simulink model "HevP4OptimalController"  (R2023b)
settings: Solver=FixedStepDiscrete  StartTime=0  StopTime=inf  FixedStep=0.01  RelTol=1e-3  EnableMultiTasking=on
model workspace (MAT data in the model file):
  AccPwrbp = Simulink.Parameter
  AccPwrbp.Value = [0 0]
  AccPwrbp.DataType = 'double'
  AccPwrbp.Complexity = 'real'
  AccPwrbp.Dimensions = [1 2]
  AccSpdbp = Simulink.Parameter
  AccSpdbp.Value = [300 750]
  AccSpdbp.DataType = 'double'
  AccSpdbp.Complexity = 'real'
  AccSpdbp.Dimensions = [1 2]
  BattChrgPwrMax = Simulink.Parameter
  BattChrgPwrMax.Value = -30000
  BattChrgPwrMax.DataType = 'double'
  BattChrgPwrMax.Complexity = 'real'
  BattChrgPwrMax.Dimensions = [1 1]
  BattCurrMax = Simulink.Parameter
  BattCurrMax.Value = 150
  BattCurrMax.DataType = 'double'
  BattCurrMax.Complexity = 'real'
  BattCurrMax.Dimensions = [1 1]
  BattDischrgPwrMax = Simulink.Parameter
  BattDischrgPwrMax.Value = 46000
  BattDischrgPwrMax.DataType = 'double'
  BattDischrgPwrMax.Complexity = 'real'
  BattDischrgPwrMax.Dimensions = [1 1]
  BattTempBp = Simulink.Parameter
  BattTempBp.Value = [243.1 253.1 263.1 273.1 283.1 298.1 313.1]
  BattTempBp.DataType = 'double'
  BattTempBp.Complexity = 'real'
  BattTempBp.Dimensions = [1 7]
  BrkPrsMax = Simulink.Parameter
  BrkPrsMax.Value = 8273709
  BrkPrsMax.DataType = 'double'
  BrkPrsMax.Complexity = 'real'
  BrkPrsMax.Dimensions = [1 1]
  CapLUTBp = Simulink.Parameter
  CapLUTBp.Value = [0 0.01 0.02 0.03 0.04 0.05 0.06 0.07 0.08 0.09 0.1 0.11 0.12 0.13 0.14 0.15 0.16 0.17 0.18 0.19 0.2 0.21 0.22 0.23 0.24 0.25 0.26 0.27 0.28 0.29 0.3 0.31 0.32 0.33 0.34 0.35 0.36 0.37 0.38 0.39 0.4 0.41 0.42 0.43 0.44 0.45 0.46 0.47 0.48 0.49 0.5 0.51 0.52 0.53 0.54 0.55 0.56 0.57 0.58 0.59 0.6 0.61 0.62 0.63 0.64 0.65 0.66 0.67 0.68 0.69 0.7 0.71 0.72 0.73 0.74 0.75 0.76 0.77 0.78 0.79 0.8 0.81 0.82 0.83 0.84 0.85 0.86 0.87 0.88 0.89 0.9 0.91 0.92 0.93 0.94 0.95 0.96 0.97 0.98 0.99 1]
  CapLUTBp.DataType = 'double'
  CapLUTBp.Complexity = 'real'
  CapLUTBp.Dimensions = [1 101]
  CapSOCBp = Simulink.Parameter
  CapSOCBp.Value = [0 0.2 0.4 0.6 0.8 1]
  CapSOCBp.DataType = 'double'
  CapSOCBp.Complexity = 'real'
  CapSOCBp.Dimensions = [1 6]
  ChrgLmt_bpt = Simulink.Parameter
  ChrgLmt_bpt.Value = [1 1 1 1 1 1 1 0.9 0.7 0.5 0]
  ChrgLmt_bpt.DataType = 'double'
  ChrgLmt_bpt.Complexity = 'real'
  ChrgLmt_bpt.Dimensions = [1 11]
  DischrgLmt_bpt = Simulink.Parameter
  DischrgLmt_bpt.Value = [0 0.5 0.7 0.9 1 1 1 1 1 1 1]
  DischrgLmt_bpt.DataType = 'double'
  DischrgLmt_bpt.Complexity = 'real'
  DischrgLmt_bpt.Dimensions = [1 11]
  ECMS_Ki = Simulink.Parameter
  ECMS_Ki.Value = 0.1
  ECMS_Ki.DataType = 'double'
  ECMS_Ki.Complexity = 'real'
  ECMS_Ki.Dimensions = [1 1]
  ECMS_Kp = Simulink.Parameter
  ECMS_Kp.Value = 3
  ECMS_Kp.DataType = 'double'
  ECMS_Kp.Complexity = 'real'
  ECMS_Kp.Dimensions = [1 1]
  ECMS_method = Simulink.Parameter
  ECMS_method.Value = 1
  ECMS_method.DataType = 'double'
  ECMS_method.Complexity = 'real'
  ECMS_method.Dimensions = [1 1]
  ECMS_s = Simulink.Parameter
  ECMS_s.Value = 3.65
  ECMS_s.DataType = 'double'
  ECMS_s.Complexity = 'real'
  ECMS_s.Dimensions = [1 1]
  Em = Simulink.Parameter
  Em.Value = [2.8 3.228 3.284 3.361 3.408 3.427 3.472 3.477 3.493 3.504 3.516 3.528 3.537 3.545 3.555 3.561 3.566 3.576 3.587 3.589 3.594 3.6 3.608 3.61 3.616 3.619 3.626 3.632 3.637 3.64 3.645 3.646 3.652 3.655 3.658 3.661 3.664 3.668 3.673 3.678 3.68 3.681 3.686 3.692 3.699 3.702 3.705 3.71 3.717 3.723 3.728 3.733 3.735 3.742 3.749 3.755 3.761 3.768 3.773 3.78 3.791 3.798 3.798 3.814 3.818 3.825 3.841 3.846 3.855 3.863 3.877 3.885 3.894 3.907 3.919 3.926 3.935 3.944 3.954 3.964 3.974 3.988 3.998 4.014 4.029 4.034 4.047 4.065 4.074 4.086 4.097 4.131 4.126 4.138 4.15 4.18 4.174 4.187 4.207 4.231 4.221]
  Em.DataType = 'double'
  Em.Complexity = 'real'
  Em.Dimensions = [1 101]
  G = Simulink.Parameter
  G.Value = [0 1 2 3 4 5 6]
  G.DataType = 'double'
  G.Complexity = 'real'
  G.Dimensions = [1 7]
  HEVEngTrq_min = Simulink.Parameter
  HEVEngTrq_min.Value = 16.186104388
  HEVEngTrq_min.DataType = 'double'
  HEVEngTrq_min.Complexity = 'real'
  HEVEngTrq_min.Dimensions = [1 1]
  Lhv = Simulink.Parameter
  Lhv.Value = 46000000
  Lhv.DataType = 'double'
  Lhv.Complexity = 'real'
  Lhv.Dimensions = [1 1]
  N = Simulink.Parameter
  N.Value = [1 4.212 2.637 1.8 1.386 1 0.772]
  N.DataType = 'double'
  N.Complexity = 'real'
  N.Dimensions = [1 7]
  N_P0 = 0.001
  N_idle = Simulink.Parameter
  N_idle.Value = 750
  N_idle.DataType = 'double'
  N_idle.Complexity = 'real'
  N_idle.Dimensions = [1 1]
  Ndiff = Simulink.Parameter
  Ndiff.Value = 3.32
  Ndiff.DataType = 'double'
  Ndiff.Complexity = 'real'
  Ndiff.Dimensions = [1 1]
  Ndiff_P4 = Simulink.Parameter
  Ndiff_P4.Value = 4.1
  Ndiff_P4.DataType = 'double'
  Ndiff_P4.Complexity = 'real'
  Ndiff_P4.Dimensions = [1 1]
  Ngrid = Simulink.Parameter
  Ngrid.Value = 200
  Ngrid.DataType = 'double'
  Ngrid.Complexity = 'real'
  Ngrid.Dimensions = [1 1]
  Np = Simulink.Parameter
  Np.Value = 1
  Np.DataType = 'double'
  Np.Complexity = 'real'
  Np.Dimensions = [1 1]
  Ns = Simulink.Parameter
  Ns.Value = 72
  Ns.DataType = 'double'
  Ns.Complexity = 'real'
  Ns.Dimensions = [1 1]
  PenaltyFctr = Simulink.Parameter
  PenaltyFctr.Value = 10000000
  PenaltyFctr.DataType = 'double'
  PenaltyFctr.Complexity = 'real'
  PenaltyFctr.Dimensions = [1 1]
  RInt = Simulink.Parameter
  RInt.Value = [0.008846  0.009319  0.009027  0.00847  0.01032  0.01314; 0.006389  0.006554  0.005553  0.005525  0.006043  0.007805; 0.004364  0.004101  0.00406  0.003452  0.003846  0.004517; 0.002031  0.002563  0.002532  0.00246  0.002716  0.003047; 0.001443  0.001825  0.001795  0.001778  0.001924  0.002234; 0.0005603  0.0007192  0.0006887  0.0007557  0.0007355  0.001014; 0.001028  0.001338  0.001  0.001536  0.001546  0.002789]
  RInt.DataType = 'double'
  RInt.Complexity = 'real'
  RInt.Dimensions = [7 6]
  Re = Simulink.Parameter
  Re.Value = 0.327
  Re.DataType = 'double'
  Re.Complexity = 'real'
  Re.Dimensions = [1 1]
  RegenBrkCutOff = Simulink.Parameter
  RegenBrkCutOff.Value = [0 1]
  RegenBrkCutOff.DataType = 'double'
  RegenBrkCutOff.Complexity = 'real'
  RegenBrkCutOff.Dimensions = [1 2]
  RegenBrkSpd_bpt = Simulink.Parameter
  RegenBrkSpd_bpt.Value = [2.2352 4.4704]
  RegenBrkSpd_bpt.DataType = 'double'
  RegenBrkSpd_bpt.Complexity = 'real'
  RegenBrkSpd_bpt.Dimensions = [1 2]
  Rm = Simulink.Parameter
  Rm.Value = 0.15
  Rm.DataType = 'double'
  Rm.Complexity = 'real'
  Rm.Dimensions = [1 1]
  SOCTrgt = Simulink.Parameter
  SOCTrgt.Value = 60
  SOCTrgt.DataType = 'double'
  SOCTrgt.Complexity = 'real'
  SOCTrgt.Dimensions = [1 1]
  SOC_bpt = Simulink.Parameter
  SOC_bpt.Value = [0 0.1 0.2 0.3 0.4 0.5 0.6 0.7 0.8 0.9 1]
  SOC_bpt.DataType = 'double'
  SOC_bpt.Complexity = 'real'
  SOC_bpt.Dimensions = [1 11]
  SOCmax = Simulink.Parameter
  SOCmax.Value = 80
  SOCmax.DataType = 'double'
  SOCmax.Complexity = 'real'
  SOCmax.Dimensions = [1 1]
  SOCmin = Simulink.Parameter
  SOCmin.Value = 40
  SOCmin.DataType = 'double'
  SOCmin.Complexity = 'real'
  SOCmin.Dimensions = [1 1]
  T = Simulink.Parameter
  T.Value = 300
  T.DataType = 'double'
  T.Complexity = 'real'
  T.Dimensions = [1 1]
  T_eff_bp = Simulink.Parameter
  T_eff_bp.Value = [0 20 40 60 80 100 120 140 160 180 200]
  T_eff_bp.DataType = 'double'
  T_eff_bp.Complexity = 'real'
  T_eff_bp.Dimensions = [1 11]
  T_eff_bp_P0 = Simulink.Parameter
  T_eff_bp_P0.Value = [5.30516476973 5.78745247607 6.36619772368 7.07355302631 7.95774715459 9.09456817668 10.6103295395 12.7323954474 15.9154943092 21.2206590789 66.6666666667]
  T_eff_bp_P0.DataType = 'double'
  T_eff_bp_P0.Complexity = 'real'
  T_eff_bp_P0.Dimensions = [1 11]
  T_t = Simulink.Parameter
  T_t.Value = [200 200 200 200 190.9859317 143.2394488 114.591559 95.49296586 81.85111359 71.61972439 63.66197724 57.29577951 52.08707228 47.74648293]
  T_t.DataType = 'double'
  T_t.Complexity = 'real'
  T_t.Dimensions = [1 14]
  T_t_P0 = Simulink.Parameter
  T_t_P0.Value = [66.6666666667 66.6666666667 66.6666666667 66.6666666667 21.2206590789 15.9154943092 12.7323954474 10.6103295395 9.09456817668 7.95774715459 7.07355302631 6.36619772368 5.78745247607 5.30516476973]
  T_t_P0.DataType = 'double'
  T_t_P0.Complexity = 'real'
  T_t_P0.Dimensions = [1 14]
  Temp_bpts = Simulink.Parameter
  Temp_bpts.Value = [313 358]
  Temp_bpts.DataType = 'double'
  Temp_bpts.Complexity = 'real'
  Temp_bpts.Dimensions = [1 2]
  TracPenaltyFctr = Simulink.Parameter
  TracPenaltyFctr.Value = 50
  TracPenaltyFctr.DataType = 'double'
  TracPenaltyFctr.Complexity = 'real'
  TracPenaltyFctr.Dimensions = [1 1]
  Trq_bpts = Simulink.Parameter
  Trq_bpts.Value = [25 50 75 100 150 200 250]
  Trq_bpts.DataType = 'double'
  Trq_bpts.Complexity = 'real'
  Trq_bpts.Dimensions = [1 7]
  a = Simulink.Parameter
  a.Value = 3
  a.DataType = 'double'
  a.Complexity = 'real'
  a.Dimensions = [1 1]
  disk_abore = Simulink.Parameter
  disk_abore.Value = 0.05
  disk_abore.DataType = 'double'
  disk_abore.Complexity = 'real'
  disk_abore.Dimensions = [1 1]
  eff = Simulink.Parameter
  eff.Value = 98
  eff.DataType = 'double'
  eff.Complexity = 'real'
  eff.Dimensions = [1 1]
  efficiency_table = Simulink.Parameter
  efficiency_table.Value = [0.52  0.78  0.8  0.82  0.82  0.8  0.78  0.78  0.76  0.74  0.7; 0.52  0.78  0.8  0.82  0.82  0.8  0.78  0.78  0.76  0.74  0.7; 0.52  0.78  0.84  0.86  0.86  0.86  0.86  0.84  0.84  0.82  0.82; 0.52  0.8  0.86  0.86  0.88  0.88  0.88  0.86  0.86  0.84  0.84; 0.52  0.8  0.86  0.88  0.88  0.88  0.88  0.88  0.86  0.86  0.86; 0.52  0.8  0.86  0.88  0.9  0.9  0.9  0.9  0.88  0.88  0.88; 0.52  0.82  0.88  0.9  0.91  0.91  0.92  0.92  0.92  0.91  0.91; 0.52  0.82  0.88  0.91  0.91  0.92  0.93  0.93  0.93  0.93  0.93; 0.52  0.84  0.9  0.92  0.92  0.93  0.93  0.93  0.93  0.93  0.93; 0.62  0.86  0.91  0.93  0.93  0.93  0.93  0.93  0.93  0.93  0.93; 0.66  0.86  0.91  0.93  0.93  0.93  0.93  0.93  0.93  0.93  0.93; 0.7  0.86  0.92  0.93  0.93  0.93  0.93  0.93  0.93  0.93  0.93; 0.7  0.86  0.92  0.93  0.93  0.93  0.93  0.93  0.93  0.93  0.93; 0.72  0.86  0.91  0.93  0.93  0.93  0.93  0.93  0.93  0.93  0.93]
  efficiency_table.DataType = 'double'
  efficiency_table.Complexity = 'real'
  efficiency_table.Dimensions = [14 11]
  eta = Simulink.Parameter
  eta.Value = 1
  eta.DataType = 'double'
  eta.Complexity = 'real'
  eta.Dimensions = [1 1]
  eta_dcdc = Simulink.Parameter
  eta_dcdc.Value = 0.98
  eta_dcdc.DataType = 'double'
  eta_dcdc.Complexity = 'real'
  eta_dcdc.Dimensions = [1 1]
  eta_diff = Simulink.Parameter
  eta_diff.Value = 0.98
  eta_diff.DataType = 'double'
  eta_diff.Complexity = 'real'
  eta_diff.Dimensions = [1 1]
  eta_tbl = Simulink.Parameter
  eta_tbl.Value = [1 1 1 1 1 1 1 1 1 1 1 1 ... (1078 elements, 7x11x7x2)]
  eta_tbl.DataType = 'double'
  eta_tbl.Complexity = 'real'
  eta_tbl.Dimensions = [7 11 7 2]
  f_fuel = Simulink.Parameter
  f_fuel.Value = [0 0 0 0 0 0 0 0 0 0 0 0 ... (256 elements, 16x16)]
  f_fuel.DataType = 'double'
  f_fuel.Complexity = 'real'
  f_fuel.Dimensions = [16 16]
  f_tbrake = Simulink.Parameter
  f_tbrake.Value = [0 15 15 15 15 15 15 15 15 15 15 15 ... (256 elements, 16x16)]
  f_tbrake.DataType = 'double'
  f_tbrake.Complexity = 'real'
  f_tbrake.Dimensions = [16 16]
  f_tbrake_min = Simulink.Parameter
  f_tbrake_min.Value = [0 6.47839451267 6.81037951773 6.98724865221 7.21080756514 7.41442983108 7.6087152853 7.78836492927 7.96107212367 8.10510304828 8.24671964745 8.36469696542 8.49674350738 8.62005140167 8.74715716666 8.88039047922]
  f_tbrake_min.DataType = 'double'
  f_tbrake_min.Complexity = 'real'
  f_tbrake_min.Dimensions = [1 16]
  f_tbrake_n_bpt = Simulink.Parameter
  f_tbrake_n_bpt.Value = [0 750 1053.57142857 1357.14285714 1660.71428571 1964.28571429 2267.85714286 2571.42857143 2875 3178.57142857 3482.14285714 3785.71428571 4089.28571429 4392.85714286 4696.42857143 5000]
  f_tbrake_n_bpt.DataType = 'double'
  f_tbrake_n_bpt.Complexity = 'real'
  f_tbrake_n_bpt.Dimensions = [1 16]
  f_tbrake_t_bpt = Simulink.Parameter
  f_tbrake_t_bpt.Value = [0 15 26.4285714286 37.8571428571 49.2857142857 60.7142857143 72.1428571429 83.5714285714 95 106.428571429 117.857142857 129.285714286 140.714285714 152.142857143 163.571428571 175]
  f_tbrake_t_bpt.DataType = 'double'
  f_tbrake_t_bpt.Complexity = 'real'
  f_tbrake_t_bpt.Dimensions = [1 16]
  mu_kinetic = Simulink.Parameter
  mu_kinetic.Value = 0.35
  mu_kinetic.DataType = 'double'
  mu_kinetic.Complexity = 'real'
  mu_kinetic.Dimensions = [1 1]
  num_pads = Simulink.Parameter
  num_pads.Value = 2
  num_pads.DataType = 'double'
  num_pads.Complexity = 'real'
  num_pads.Dimensions = [1 1]
  omega_bpts = Simulink.Parameter
  omega_bpts.Value = [500.383141081 749.619781963 1002.67614148 1250.9578527 1499.23956393 1747.52127515 1995.80298637 2501.9157054 2998.47912785 4001.15526933 5003.83141081]
  omega_bpts.DataType = 'double'
  omega_bpts.Complexity = 'real'
  omega_bpts.Dimensions = [1 11]
  w_eff_bp = Simulink.Parameter
  w_eff_bp.Value = [0 500 1000 1432.391138 1500 2000 2500 3000 3500 4000 4500 5000 5500 6000]
  w_eff_bp.DataType = 'double'
  w_eff_bp.Complexity = 'real'
  w_eff_bp.Dimensions = [1 14]
  w_eff_bp_P0 = Simulink.Parameter
  w_eff_bp_P0.Value = [0 500 1000 1432.39448783 4500 6000 7500 9000 10500 12000 13500 15000 16500 18000]
  w_eff_bp_P0.DataType = 'double'
  w_eff_bp_P0.Complexity = 'real'
  w_eff_bp_P0.Dimensions = [1 14]
libraries: simulink x3, autolibhevctrlrcommon x2, autolibhevctrlr x1
settings Model: DataDictionary=HevP4OptimalController.sldd  ModifiedByFormat=The MathWorks, Inc.  Creator=The MathWorks, Inc.  LastModifiedBy=The MathWorks, Inc.
settings SolverCC: AlgebraicLoopSolver=TrustRegion  MaxZcPerStep=1
settings DataIOCC: SaveOutput=off  SignalLogging=off  DSMLogging=off  SaveTime=off  ReturnWorkspaceOutputs=off
settings OptimizationCC: DefaultParameterBehavior=Inlined  EnhancedBackFolding=on  PassReuseOutputArgsAs=Individual arguments  ZeroExternalMemoryAtStartup=off  ZeroInternalMemoryAtStartup=off  EfficientMapNaN2IntZero=off  OptimizeBlockOrder=speed  DifferentSizesBufferReuse=on  OptimizationCustomize=off  EfficientTunableParamExpr=on
settings DebuggingCC: UnderspecifiedInitializationDetection=Classic  MergeDetectMultiDrivingBlocksExec=none  ParameterTunabilityLossMsg=error  UnconnectedInputMsg=warning  UnconnectedOutputMsg=warning  UnconnectedLineMsg=warning  SubsystemReferenceDiagnosticForUnitTest=warning  SFUnusedDataAndEventsDiag=none  ArithmeticOperatorsInVariantConditions=warning
settings HardwareCC: TargetBitPerPointer=64  TargetBitPerSizeT=64  TargetBitPerPtrDiffT=64  TargetLongLongMode=on  TargetIntDivRoundTo=Zero  TargetEndianess=LittleEndian  TargetWordSize=64  TargetHWDeviceType=MATLAB Host  ProdEqTarget=off
settings ModelReferenceCC: EnableRefExpFcnMdlSchedulingChecks=on
settings SFSimCC: SimUseLocalCustomCode=off  SimGenImportedTypeDefs=on  MATLABDynamicMemAlloc=off
settings RTWCC: Description=AUTOSAR  SystemTargetFile=autosar.tlc  GenCodeOnly=on  TemplateMakefile=ert_default_tmf  RTWUseLocalCustomCode=off  DLArmComputeVersion=19.05
settings CodeAppCC: ForceParamTrailComments=on  IgnoreCustomStorageClasses=off  MaxIdLength=128  OperatorAnnotations=on  SimulinkDataObjDesc=on  SFDataObjDesc=on  InsertBlockDesc=on
settings STFCustomTargetCC: TargetLangStandard=C89/C90 (ANSI)  MultiwordLength=256  ParMdlRefBuildCompliant=on  CompOptLevelCompliant=on  IncludeMdlTerminateFcn=off  CombineOutputUpdateFcns=on  SuppressErrorStatus=on  ERTCustomFileBanners=on  SupportNonFinite=off  SupportComplex=off  SupportContinuousTime=off  SupportNonInlinedSFcns=off  RemoveResetFunc=on  MATLABClassNameForMDSCustomization=Simulink.SoftwareTarget.ERTCustomization  AutosarCompliant=on  UseToolchainInfoCompliant=on  LookupTableObjectStructAxisOrder=2,1,3,4,...  LUTObjectStructOrderEvenSpacing=Size,Table,Breakpoints  SystemTargetFile=autosar.tlc
settings ERTTargetCC: ConcurrentExecutionCompliant=off  IncludeMdlTerminateFcn=off  SuppressErrorStatus=on  SupportNonFinite=off  SupportComplex=off  ModelStepFunctionPrototypeControlCompliant=off  CPPClassGenCompliant=off  AutosarCompliant=on  LookupTableObjectStructAxisOrder=2,1,3,4,...  LUTObjectStructOrderEvenSpacing=Size,Table,Breakpoints  InlinedParameterPlacement=NonHierarchical  ERTCustomFileTemplate=example_file_process.tlc
settings ConfigComp: CovMetricSettings=dsw  CovSaveCumulativeToWorkspaceVar=on  CovSaveSingleToWorkspaceVar=on  CovExternalEMLEnable=off

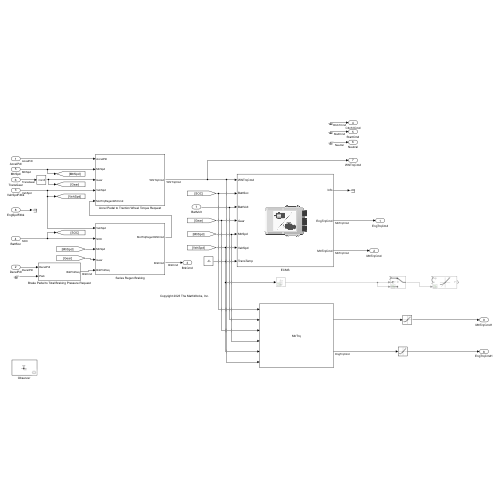
[thumbnail: Simulink's stored preview of the top-level diagram]
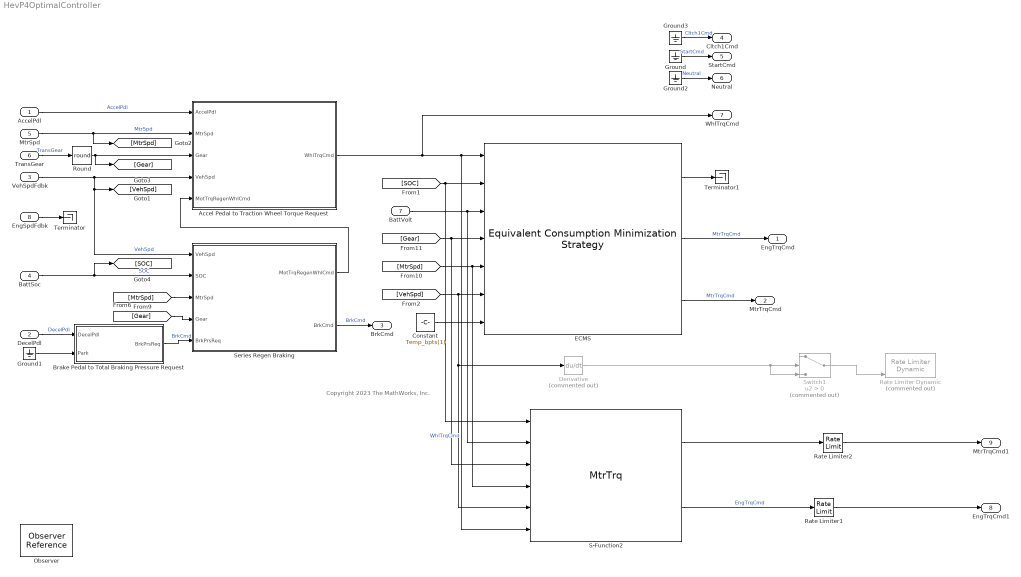
== system HevP4OptimalController ==
  note: Copyright 2023 The MathWorks, Inc.
  AccelPdl : Inport  OutDataTypeStr=double  PortDimensions=1  SampleTime=[0.01,0]
  DecelPdl : Inport  Port=2  OutDataTypeStr=double  PortDimensions=1  SampleTime=[0.01,0]
  VehSpdFdbk : Inport  Port=3  OutDataTypeStr=double  PortDimensions=1  SampleTime=[0.01,0]
  BattSoc : Inport  Port=4  OutDataTypeStr=double  PortDimensions=1  SampleTime=[0.01,0]
  MtrSpd : Inport  Port=5  OutDataTypeStr=double  PortDimensions=1  SampleTime=[0.01,0]
  TransGear : Inport  Port=6  OutDataTypeStr=double  PortDimensions=1  SampleTime=[0.01,0]
  BattVolt : Inport  Port=7  OutDataTypeStr=double  PortDimensions=1  SampleTime=[0.01,0]
  EngSpdFdbk : Inport  Port=8  OutDataTypeStr=double  PortDimensions=1  SampleTime=[0.01,0]
  Accel Pedal to Traction Wheel Torque Request : Subsystem
  Brake Pedal to Total Braking Pressure Request : Subsystem
  Constant : Constant  Value=Temp_bpts(1)
  Derivative : Derivative  Commented=on
  ECMS : autolibhevctrlr/Equivalent Consumption Minimization Strategy  HevMtrLoc=P4  EcmsMethod=Non-adaptive  N_diff=Ndiff  eta_diff=eta_diff  N_diff_P4=Ndiff_P4  Re=Re  TransEffFactors=Gear, input torque, input speed, and temperature  G_trans=G  N_trans=N  Trq_trans_bpts=Trq_bpts  omega_trans_bpts=omega_bpts  Temp_trans_bpts=Temp_bpts  eta_trans=[1 1 1 1 1 1 1]  eta_trans_tbl=eta_tbl  f_tbrake_n_bpt=f_tbrake_n_bpt  f_tbrake_t_bpt=f_tbrake_t_bpt  f_tbrake=f_tbrake  f_tbrake_min=f_tbrake_min  f_fuel=f_fuel  HEVEngTrq_min=HEVEngTrq_min  LHV=Lhv  AccPwrTbl=AccPwrbp  AccSpdBpts=AccSpdbp  N_idle=N_idle  SOC_bpt=SOC_bpt  ChrgLmt=ChrgLmt_bpt  DischrgLmt=DischrgLmt_bpt  BattCurrMax=BattCurrMax  eta_dcdc=eta_dcdc  BattChrgPwrMax=BattChrgPwrMax  BattDischrgPwrMax=BattDischrgPwrMax  MtrEffiMethod=Positive speed and full torque range  f_tmtr_max=T_t  f_mtr_w_bpt=w_eff_bp  f_mtr_t_bpt=T_eff_bp  f_mtr_eta=efficiency_table  Ngrid=Ngrid  N_P0=N_P0  ECMS_s=ECMS_s  a=a  ECMS_Kp=ECMS_Kp  ECMS_Ki=ECMS_Ki  PenaltyFctr=PenaltyFctr  SOCTrgt=SOCTrgt  SOCmin=SOCmin  SOCmax=SOCmax
  Ground{,1..3} (4 alike) : Ground
  Observer : ObserverReference  ObserverModelName=HevP4OptimalController_Observer1
  Rate Limiter Dynamic : simulink/Discontinuities/Rate Limiter Dynamic  Commented=on
  Rate Limiter1 : RateLimiter  RisingSlewLimit=80  FallingSlewLimit=-30  SampleTimeMode=inherited
  Rate Limiter2 : RateLimiter  RisingSlewLimit=55  FallingSlewLimit=-55  SampleTimeMode=inherited
  Round : Rounding  Operator=round
  S-Function2 : S-Function  FunctionName=MtrTrq  SFunctionDeploymentMode=off  EnableBusSupport=off
  Series Regen Braking : Subsystem  VariantControl=0
  Switch1 : Switch  Commented=on  Criteria=u2 > Threshold  SaturateOnIntegerOverflow=off  InputSameDT=off
  Terminator : Terminator
  Terminator1 : Terminator
  EngTrqCmd : Outport  OutDataTypeStr=double  PortDimensions=1  SampleTime=[0.01,0]  VectorParamsAs1DForOutWhenUnconnected=off
  MtrTrqCmd : Outport  Port=2  OutDataTypeStr=double  PortDimensions=1  SampleTime=[0.01,0]  VectorParamsAs1DForOutWhenUnconnected=off
  BrkCmd : Outport  Port=3  OutDataTypeStr=double  PortDimensions=1  SampleTime=[0.01,0]  VectorParamsAs1DForOutWhenUnconnected=off
  Cltch1Cmd : Outport  Port=4  PortDimensions=1  SampleTime=[0.01,0]  VectorParamsAs1DForOutWhenUnconnected=off
  StartCmd : Outport  Port=5  PortDimensions=1  SampleTime=[0.01,0]  VectorParamsAs1DForOutWhenUnconnected=off
  Neutral : Outport  Port=6  PortDimensions=1  SampleTime=[0.01,0]  VectorParamsAs1DForOutWhenUnconnected=off
  WhlTrqCmd : Outport  Port=7  OutDataTypeStr=double  PortDimensions=1  SampleTime=[0.01,0]  VectorParamsAs1DForOutWhenUnconnected=off
  EngTrqCmd1 : Outport  Port=8  OutDataTypeStr=double  PortDimensions=1  SampleTime=[0.01,0]  VectorParamsAs1DForOutWhenUnconnected=off
  MtrTrqCmd1 : Outport  Port=9  OutDataTypeStr=double  PortDimensions=1  SampleTime=[0.01,0]  VectorParamsAs1DForOutWhenUnconnected=off
  wires:
  AccelPdl/1 -> Accel Pedal to Traction Wheel Torque Request/1(AccelPdl)  "AccelPdl"
  DecelPdl/1 -> Brake Pedal to Total Braking Pressure Request/1(DecelPdl)  "DecelPdl"
  VehSpdFdbk/1 -> Series Regen Braking/1(VehSpd), [VehSpd], Accel Pedal to Traction Wheel Torque Request/4(VehSpd)  "VehSpd"
  [SOC] -> S-Function2/1, ECMS/2
  MtrSpd/1 -> [MtrSpd], Accel Pedal to Traction Wheel Torque Request/2(MtrSpd)  "MtrSpd"
  Accel Pedal to Traction Wheel Torque Request/1(WhlTrqCmd) -> WhlTrqCmd/1, ECMS/1, S-Function2/6  "WhlTrqCmd"
  Series Regen Braking/2(" BrkCmd") -> BrkCmd/1  "BrkCmd"
  Ground1/1 -> Brake Pedal to Total Braking Pressure Request/2(Park)
  TransGear/1 -> Round/1  "TransGear"
  Ground3/1 -> Cltch1Cmd/1  "Cltch1Cmd"
  Brake Pedal to Total Braking Pressure Request/1(BrkPrsReq) -> Series Regen Braking/5("BrkPrsReq ")  "BrkCmd"
  Series Regen Braking/1(" MotTrqRegenWhlCmd") -> Accel Pedal to Traction Wheel Torque Request/5(MotTrqRegenWhlCmd)
  [MtrSpd] -> Series Regen Braking/3(MtrSpd)
  [Gear] -> Series Regen Braking/4(Gear)
  Ground/1 -> StartCmd/1  "StartCmd"
  Ground2/1 -> Neutral/1  "Neutral"
  EngSpdFdbk/1 -> Terminator/1
  [Gear] -> S-Function2/3, ECMS/4
  [VehSpd] -> S-Function2/5, Derivative/1, ECMS/6
  Constant/1 -> ECMS/7
  BattSoc/1 -> [SOC], Series Regen Braking/2(SOC)  "SOC"
  Round/1 -> [Gear], Accel Pedal to Traction Wheel Torque Request/3(Gear)
  ECMS/1 -> Terminator1/1
  ECMS/3 -> MtrTrqCmd/1  "MtrTrqCmd"
  ECMS/2 -> EngTrqCmd/1  "MtrTrqCmd"
  BattVolt/1 -> ECMS/3, S-Function2/2
  [MtrSpd] -> S-Function2/4, ECMS/5
  Derivative/1 -> Switch1/3, Switch1/2
  Switch1/1 -> Rate Limiter Dynamic/3
  S-Function2/1 -> Rate Limiter2/1
  S-Function2/2 -> Rate Limiter1/1  "EngTrqCmd"
  Rate Limiter2/1 -> MtrTrqCmd1/1
  Rate Limiter1/1 -> EngTrqCmd1/1

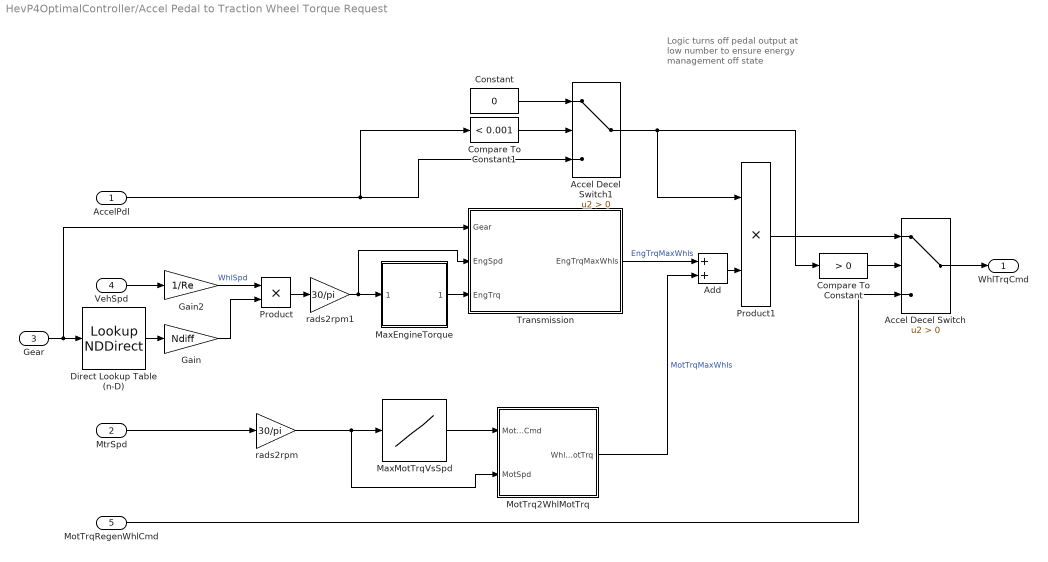
== system HevP4OptimalController/Accel Pedal to Traction Wheel Torque Request ==
  note: Logic turns off pedal
      | output at low number
      | to ensure energy
      | management off state
  AccelPdl : Inport
  MtrSpd : Inport  Port=2
  Gear : Inport  Port=3
  VehSpd : Inport  Port=4
  MotTrqRegenWhlCmd : Inport  Port=5
  Accel Decel Switch : Switch  Criteria=u2 > Threshold  SaturateOnIntegerOverflow=off  InputSameDT=off
  Accel Decel Switch1 : Switch  Criteria=u2 > Threshold  SaturateOnIntegerOverflow=off  InputSameDT=off
  Add : Sum
  Compare To Constant : simulink/Logic and Bit Operations/Compare To Constant  relop=>  const=0  OutDataTypeStr=boolean
  Compare To Constant1 : simulink/Logic and Bit Operations/Compare To Constant  relop=<  const=0.001  OutDataTypeStr=boolean
  Constant : Constant  Value=0
  Direct Lookup Table (n-D) : LookupNDDirect  NumberOfTableDimensions=1  Table=N
  Gain : Gain  Gain=Ndiff
  Gain2 : Gain  Gain=1/Re
  MaxEngineTorque : Subsystem
  MaxMotTrqVsSpd : Lookup_n-D  NumberOfTableDimensions=1  BreakpointsForDimension1=w_eff_bp  Table=T_t  ExtrapMethod=Clip  UseLastTableValue=on  InternalRulePriority=Speed  OutDataTypeStr=Inherit: Inherit from 'Table data'  RndMeth=Simplest
  MotTrq2WhlMotTrq : Subsystem  VariantControl=3
  Product : Product
  Product1 : Product
  Transmission : Subsystem
  rads2rpm : Gain  Gain=30/pi
  rads2rpm1 : Gain  Gain=30/pi
  WhlTrqCmd : Outport  VectorParamsAs1DForOutWhenUnconnected=off
  wires:
  AccelPdl/1 -> Compare To Constant1/1, Accel Decel Switch1/3
  MaxEngineTorque/1(EngTrq) -> Transmission/3(EngTrq)
  MaxMotTrqVsSpd/1 -> MotTrq2WhlMotTrq/1(MotTrqCmd)
  rads2rpm/1 -> MotTrq2WhlMotTrq/2(MotSpd), MaxMotTrqVsSpd/1
  MtrSpd/1 -> rads2rpm/1
  Gear/1 -> Transmission/1(Gear), Direct Lookup Table (n-D)/1
  MotTrqRegenWhlCmd/1 -> Accel Decel Switch/3
  Compare To Constant/1 -> Accel Decel Switch/2
  Product1/1 -> Accel Decel Switch/1
  Accel Decel Switch/1 -> WhlTrqCmd/1
  MotTrq2WhlMotTrq/1(WhlMotTrq) -> Add/2  "MotTrqMaxWhls"
  VehSpd/1 -> Gain2/1
  Gain2/1 -> Product/1  "WhlSpd"
  Gain/1 -> Product/2
  Product/1 -> rads2rpm1/1
  rads2rpm1/1 -> MaxEngineTorque/1(EngSpd), Transmission/2(EngSpd)
  Direct Lookup Table (n-D)/1 -> Gain/1
  Transmission/1(EngTrqMaxWhls) -> Add/1  "EngTrqMaxWhls"
  Add/1 -> Product1/2
  Compare To Constant1/1 -> Accel Decel Switch1/2
  Accel Decel Switch1/1 -> Product1/1, Compare To Constant/1
  Constant/1 -> Accel Decel Switch1/1

== system HevP4OptimalController/Brake Pedal to Total Braking Pressure Request ==
  DecelPdl : Inport
  Park : Inport  Port=2
  Constant : Constant  Value=BrkPrsMax
  Constant1 : Constant
  Product1 : Product
  Switch : Switch  Criteria=u2 > Threshold  SaturateOnIntegerOverflow=off  InputSameDT=off
  BrkPrsReq : Outport  VectorParamsAs1DForOutWhenUnconnected=off
  wires:
  Constant/1 -> Product1/2
  Switch/1 -> Product1/1
  DecelPdl/1 -> Switch/3
  Constant1/1 -> Switch/1
  Product1/1 -> BrkPrsReq/1
  Park/1 -> Switch/2

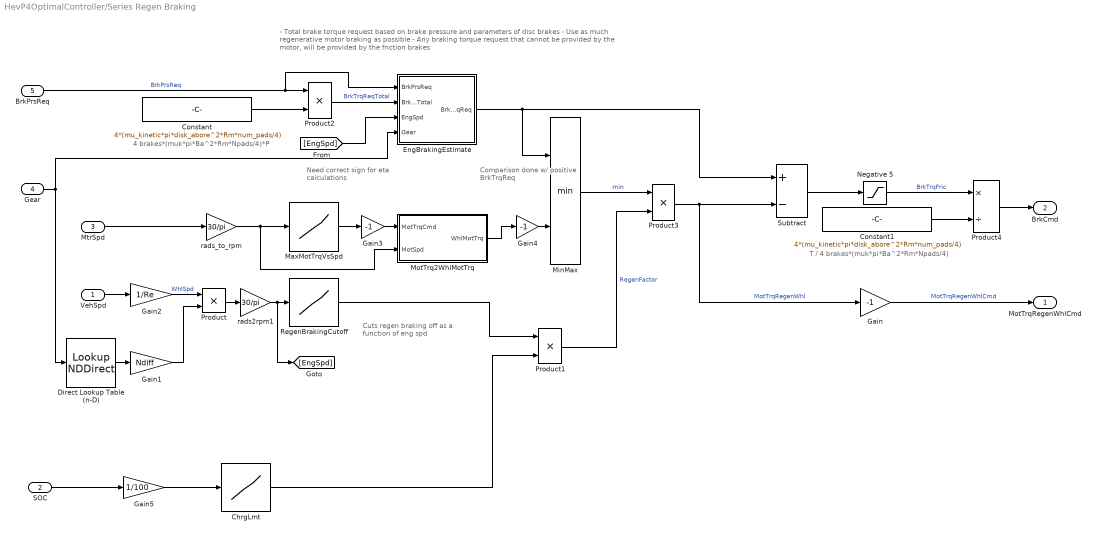
== system HevP4OptimalController/Series Regen Braking ==
  note: Comparison done
      | w/ positive BrkTrqReq
  note: Need correct sign
      | for eta calculations
  note: Cuts regen braking off
      | as a function of eng spd
  note: - Total brake torque request based on brake pressure and parameters of disc brakes
      | - Use as much regenerative motor braking as possible
      | -  Any braking torque request that cannot be provided by the motor, will be provided by the friction brakes
  note: T / 4 brakes*(muk*pi*Ba^2*Rm*Npads/4)
  note: 4 brakes*(muk*pi*Ba^2*Rm*Npads/4)*P
  VehSpd : Inport
  SOC : Inport  Port=2
  MtrSpd : Inport  Port=3
  Gear : Inport  Port=4
  "BrkPrsReq " : Inport  Port=5
  ChrgLmt : Lookup_n-D  NumberOfTableDimensions=1  BreakpointsForDimension1=SOC_bpt  Table=ChrgLmt_bpt  ExtrapMethod=Clip  UseLastTableValue=on  InternalRulePriority=Speed  RndMeth=Simplest
  Constant : Constant  Value=4*(mu_kinetic*pi*disk_abore^2*Rm*num_pads/4)
  Constant1 : Constant  Value=4*(mu_kinetic*pi*disk_abore^2*Rm*num_pads/4)
  Direct Lookup Table (n-D) : LookupNDDirect  NumberOfTableDimensions=1  Table=N
  EngBrakingEstimate : Subsystem
  Gain : Gain  Gain=-1
  Gain1 : Gain  Gain=Ndiff
  Gain2 : Gain  Gain=1/Re
  Gain3 : Gain  Gain=-1
  Gain4 : Gain  Gain=-1
  Gain5 : Gain  Gain=1/100
  MaxMotTrqVsSpd : Lookup_n-D  NumberOfTableDimensions=1  BreakpointsForDimension1=w_eff_bp  Table=T_t  ExtrapMethod=Clip  UseLastTableValue=on  InternalRulePriority=Speed  OutDataTypeStr=Inherit: Inherit from 'Table data'  RndMeth=Simplest
  MinMax : MinMax  Inputs=2
  MotTrq2WhlMotTrq : Subsystem  VariantControl=3
  Negative 5 : Saturate  UpperLimit=inf  LowerLimit=0
  Product{,1..3} (4 alike) : Product
  Product4 : Product  Inputs=*/
  RegenBrakingCutoff : Lookup_n-D  NumberOfTableDimensions=1  BreakpointsForDimension1=[f_tbrake_n_bpt(2) f_tbrake_n_bpt(3)]  Table=RegenBrkCutOff  ExtrapMethod=Clip  UseLastTableValue=on  InternalRulePriority=Speed  RndMeth=Simplest
  Subtract : Sum  Inputs=+-
  rads2rpm1 : Gain  Gain=30/pi
  rads_to_rpm : Gain  Gain=30/pi
  " MotTrqRegenWhlCmd" : Outport  VectorParamsAs1DForOutWhenUnconnected=off
  " BrkCmd" : Outport  Port=2  VectorParamsAs1DForOutWhenUnconnected=off
  wires:
  Product3/1 -> Gain/1, Subtract/2  "MotTrqRegenWhl"
  Product4/1 -> " BrkCmd"/1
  Constant1/1 -> Product4/2
  Constant/1 -> Product2/2
  "BrkPrsReq "/1 -> EngBrakingEstimate/1(BrkPrsReq), Product2/1  "BrkPrsReq"
  rads_to_rpm/1 -> MotTrq2WhlMotTrq/2(MotSpd), MaxMotTrqVsSpd/1
  Gain3/1 -> MotTrq2WhlMotTrq/1(MotTrqCmd)
  MinMax/1 -> Product3/1  "min"
  RegenBrakingCutoff/1 -> Product1/1
  Subtract/1 -> Negative 5/1
  Negative 5/1 -> Product4/1  "BrkTrqFric"
  MtrSpd/1 -> rads_to_rpm/1
  MotTrq2WhlMotTrq/1(WhlMotTrq) -> Gain4/1
  Gain/1 -> " MotTrqRegenWhlCmd"/1  "MotTrqRegenWhlCmd"
  Gear/1 -> Direct Lookup Table (n-D)/1, EngBrakingEstimate/4(Gear)
  Gain1/1 -> Product/2
  Product/1 -> rads2rpm1/1
  Direct Lookup Table (n-D)/1 -> Gain1/1
  VehSpd/1 -> Gain2/1
  Gain2/1 -> Product/1  "WhlSpd"
  rads2rpm1/1 -> [EngSpd], RegenBrakingCutoff/1
  MaxMotTrqVsSpd/1 -> Gain3/1
  Gain4/1 -> MinMax/2
  EngBrakingEstimate/1(BrkTrqReq) -> Subtract/1, MinMax/1
  Product2/1 -> EngBrakingEstimate/2(BrkTrqReqTotal)  "BrkTrqReqTotal"
  [EngSpd] -> EngBrakingEstimate/3(EngSpd)
  ChrgLmt/1 -> Product1/2
  Gain5/1 -> ChrgLmt/1
  SOC/1 -> Gain5/1
  Product1/1 -> Product3/2  "RegenFactor"

== system HevP4OptimalController/Accel Pedal to Traction Wheel Torque Request/MaxEngineTorque ==
  note: Account for net torque of
      | eng due to accessory load
  EngSpd : Inport
  Accessory Load Model : autolibhevctrlrcommon/Accessory Load Model  AccPwrTbl=[0 0]  AccSpdBpts=[300 750]
  MaxEngineTorque : Lookup_n-D  NumberOfTableDimensions=1  BreakpointsForDimension1=f_tbrake_n_bpt  Table=[0 max(f_tbrake(:,2:end))]  ExtrapMethod=Clip  UseLastTableValue=on  InternalRulePriority=Speed  RndMeth=Simplest
  Minus : Sum  Inputs=+-
  EngTrq : Outport
  wires:
  MaxEngineTorque/1 -> Minus/1
  EngSpd/1 -> Accessory Load Model/1, MaxEngineTorque/1
  Accessory Load Model/1 -> Minus/2
  Minus/1 -> EngTrq/1

== system HevP4OptimalController/Accel Pedal to Traction Wheel Torque Request/MotTrq2WhlMotTrq ==
  MotTrqCmd : Inport
  MotSpd : Inport  Port=2
  Diff Eta : Subsystem
  Divide2 : Product  Inputs=**
  Gain3 : Gain  Gain=Ndiff_P4
  WhlMotTrq : Outport  VectorParamsAs1DForOutWhenUnconnected=off
  wires:
  MotTrqCmd/1 -> Diff Eta/2(TrqIn), Gain3/1
  Diff Eta/1(eta) -> Divide2/1
  Gain3/1 -> Divide2/2
  MotSpd/1 -> Diff Eta/1(SpdIn)
  Divide2/1 -> WhlMotTrq/1

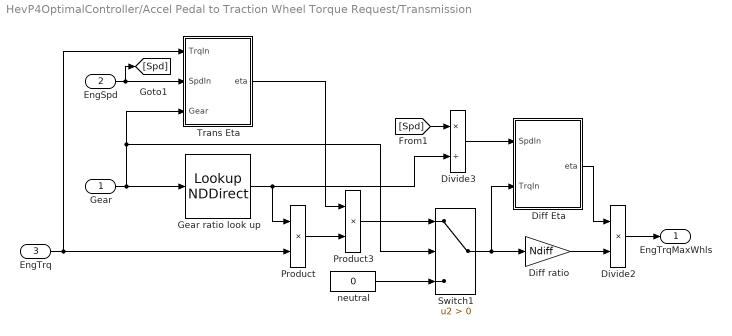
== system HevP4OptimalController/Accel Pedal to Traction Wheel Torque Request/Transmission ==
  Gear : Inport
  EngSpd : Inport  Port=2
  EngTrq : Inport  Port=3
  Diff Eta : Subsystem
  Diff ratio : Gain  Gain=Ndiff
  Divide2 : Product  Inputs=**
  Divide3 : Product  Inputs=*/
  Gear ratio look up : LookupNDDirect  NumberOfTableDimensions=1  Table=N
  Product : Product  RndMeth=Zero
  Product3 : Product  Inputs=**  RndMeth=Zero
  Switch1 : Switch  Criteria=u2 > Threshold  SaturateOnIntegerOverflow=off  InputSameDT=off
  Trans Eta : Subsystem
  neutral : Constant  Value=0
  EngTrqMaxWhls : Outport  VectorParamsAs1DForOutWhenUnconnected=off
  wires:
  Product/1 -> Product3/2
  Switch1/1 -> Diff Eta/2(TrqIn), Diff ratio/1
  Gear ratio look up/1 -> Divide3/2, Product/1
  Gear/1 -> Gear ratio look up/1, Trans Eta/3(Gear), Switch1/2
  Trans Eta/1(eta) -> Product3/1
  neutral/1 -> Switch1/3
  Product3/1 -> Switch1/1
  Diff ratio/1 -> Divide2/2
  EngSpd/1 -> [Spd], Trans Eta/2(SpdIn)
  EngTrq/1 -> Trans Eta/1(TrqIn), Product/2
  Diff Eta/1(eta) -> Divide2/1
  Divide2/1 -> EngTrqMaxWhls/1
  Divide3/1 -> Diff Eta/1(SpdIn)
  [Spd] -> Divide3/1

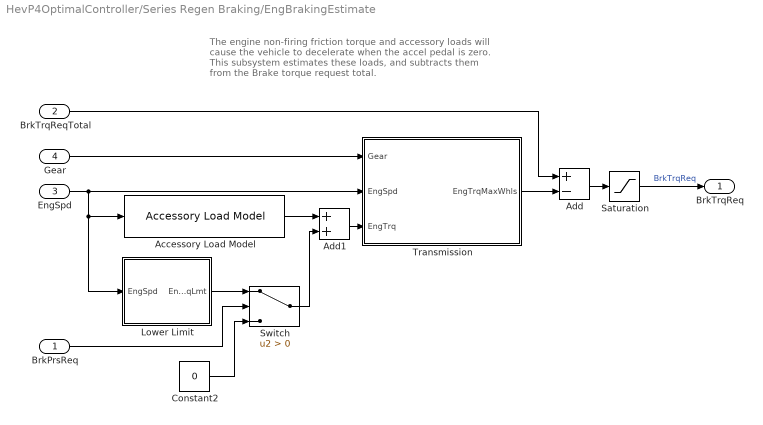
== system HevP4OptimalController/Series Regen Braking/EngBrakingEstimate ==
  note: The engine non-firing friction torque and accessory loads
      | will cause the vehicle to decelerate when the accel pedal
      | is zero.  This subsystem estimates these loads, and
      | subtracts them from the Brake torque request total.
  BrkPrsReq : Inport
  BrkTrqReqTotal : Inport  Port=2
  EngSpd : Inport  Port=3
  Gear : Inport  Port=4
  Accessory Load Model : autolibhevctrlrcommon/Accessory Load Model  AccPwrTbl=[0 0]  AccSpdBpts=[300 750]
  Add : Sum  Inputs=+-
  Add1 : Sum
  Constant2 : Constant  Value=0
  Lower Limit : Subsystem
  Saturation : Saturate  UpperLimit=inf  LowerLimit=0
  Switch : Switch  Criteria=u2 > Threshold  SaturateOnIntegerOverflow=off  InputSameDT=off
  Transmission : Subsystem
  BrkTrqReq : Outport  VectorParamsAs1DForOutWhenUnconnected=off
  wires:
  EngSpd/1 -> Accessory Load Model/1, Lower Limit/1(EngSpd), Transmission/2(EngSpd)
  Add/1 -> Saturation/1
  Switch/1 -> Add1/2
  Saturation/1 -> BrkTrqReq/1  "BrkTrqReq"
  Lower Limit/1(EngTrqLmt) -> Switch/1
  BrkTrqReqTotal/1 -> Add/1
  Accessory Load Model/1 -> Add1/1
  Constant2/1 -> Switch/3
  Add1/1 -> Transmission/3(EngTrq)
  Transmission/1(EngTrqMaxWhls) -> Add/2
  BrkPrsReq/1 -> Switch/2
  Gear/1 -> Transmission/1(Gear)

== system HevP4OptimalController/Series Regen Braking/MotTrq2WhlMotTrq ==
  MotTrqCmd : Inport
  MotSpd : Inport  Port=2
  Diff Eta : Subsystem
  Divide2 : Product  Inputs=**
  Gain3 : Gain  Gain=Ndiff_P4
  WhlMotTrq : Outport  VectorParamsAs1DForOutWhenUnconnected=off
  wires:
  MotTrqCmd/1 -> Diff Eta/2(TrqIn), Gain3/1
  Diff Eta/1(eta) -> Divide2/1
  Gain3/1 -> Divide2/2
  MotSpd/1 -> Diff Eta/1(SpdIn)
  Divide2/1 -> WhlMotTrq/1

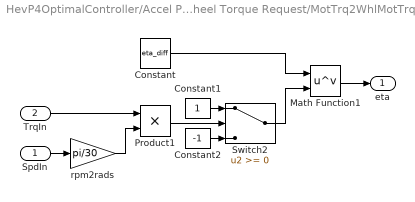
== system HevP4OptimalController/Accel Pedal to Traction Wheel Torque Request/MotTrq2WhlMotTrq/Diff Eta ==
  SpdIn : Inport
  TrqIn : Inport  Port=2
  Constant : Constant  Value=eta_diff
  Constant1 : Constant  SampleTime=-1
  Constant2 : Constant  Value=-1  SampleTime=-1
  Math Function1 : Math  Operator=pow  SignedPower=on  OutputSignalType=real
  Product1 : Product
  Switch2 : Switch  SaturateOnIntegerOverflow=off  InputSameDT=off
  rpm2rads : Gain  Gain=pi/30
  eta : Outport  VectorParamsAs1DForOutWhenUnconnected=off
  wires:
  rpm2rads/1 -> Product1/2
  Constant/1 -> Math Function1/1
  Constant2/1 -> Switch2/3
  Constant1/1 -> Switch2/1
  Product1/1 -> Switch2/2
  Switch2/1 -> Math Function1/2
  Math Function1/1 -> eta/1
  SpdIn/1 -> rpm2rads/1
  TrqIn/1 -> Product1/1

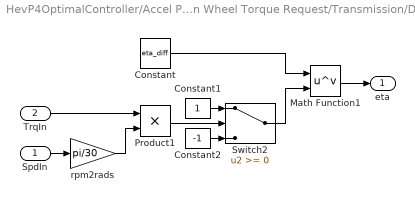
== system HevP4OptimalController/Accel Pedal to Traction Wheel Torque Request/Transmission/Diff Eta ==
  SpdIn : Inport
  TrqIn : Inport  Port=2
  Constant : Constant  Value=eta_diff
  Constant1 : Constant  SampleTime=-1
  Constant2 : Constant  Value=-1  SampleTime=-1
  Math Function1 : Math  Operator=pow  SignedPower=on  OutputSignalType=real
  Product1 : Product
  Switch2 : Switch  SaturateOnIntegerOverflow=off  InputSameDT=off
  rpm2rads : Gain  Gain=pi/30
  eta : Outport  VectorParamsAs1DForOutWhenUnconnected=off
  wires:
  rpm2rads/1 -> Product1/2
  Constant/1 -> Math Function1/1
  Constant2/1 -> Switch2/3
  Constant1/1 -> Switch2/1
  Product1/1 -> Switch2/2
  Switch2/1 -> Math Function1/2
  Math Function1/1 -> eta/1
  SpdIn/1 -> rpm2rads/1
  TrqIn/1 -> Product1/1

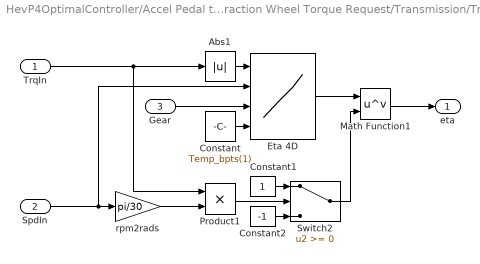
== system HevP4OptimalController/Accel Pedal to Traction Wheel Torque Request/Transmission/Trans Eta ==
  TrqIn : Inport
  SpdIn : Inport  Port=2
  Gear : Inport  Port=3
  Abs1 : Abs  SaturateOnIntegerOverflow=off
  Constant : Constant  Value=Temp_bpts(1)
  Constant1 : Constant  SampleTime=-1
  Constant2 : Constant  Value=-1  SampleTime=-1
  Eta 4D : Lookup_n-D  NumberOfTableDimensions=4  LookupTableObject=''  BreakpointsForDimension1=Trq_bpts  BreakpointsForDimension2=omega_bpts  BreakpointsForDimension3=G  BreakpointsForDimension4=Temp_bpts  Table=eta_tbl  ExtrapMethod=Clip  InternalRulePriority=Speed  RndMeth=Simplest
      settings: InputPortMap=u0,u1,u2,u3
  Math Function1 : Math  Operator=pow  SignedPower=on  OutputSignalType=real
  Product1 : Product
  Switch2 : Switch  SaturateOnIntegerOverflow=off  InputSameDT=off
  rpm2rads : Gain  Gain=pi/30
  eta : Outport  VectorParamsAs1DForOutWhenUnconnected=off
  wires:
  TrqIn/1 -> Product1/1, Abs1/1
  SpdIn/1 -> Eta 4D/2, rpm2rads/1
  Math Function1/1 -> eta/1
  Abs1/1 -> Eta 4D/1
  Switch2/1 -> Math Function1/2
  Product1/1 -> Switch2/2
  Constant1/1 -> Switch2/1
  Constant2/1 -> Switch2/3
  Eta 4D/1 -> Math Function1/1
  rpm2rads/1 -> Product1/2
  Gear/1 -> Eta 4D/3
  Constant/1 -> Eta 4D/4

== system HevP4OptimalController/Series Regen Braking/EngBrakingEstimate/Lower Limit ==
  note: Engine non-firing friction torque
      | (0 torque command row of f_tbrake map)
  EngSpd : Inport
  Gain5 : Gain  Gain=-1
  Max Torque vs Speed : Lookup_n-D  NumberOfTableDimensions=1  BreakpointsForDimension1=[0 749 f_tbrake_n_bpt(:,2:end)]  Table=[0 0 min(f_tbrake(:,2:end))]  ExtrapMethod=Clip  UseLastTableValue=on  RndMeth=Simplest
  Saturation1 : Saturate  UpperLimit=inf  LowerLimit=0
  EngTrqLmt : Outport  VectorParamsAs1DForOutWhenUnconnected=off
  wires:
  EngSpd/1 -> Max Torque vs Speed/1
  Gain5/1 -> Saturation1/1
  Max Torque vs Speed/1 -> Gain5/1
  Saturation1/1 -> EngTrqLmt/1

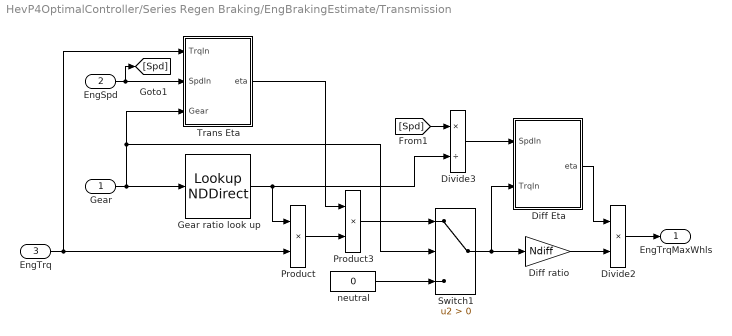
== system HevP4OptimalController/Series Regen Braking/EngBrakingEstimate/Transmission ==
  Gear : Inport
  EngSpd : Inport  Port=2
  EngTrq : Inport  Port=3
  Diff Eta : Subsystem
  Diff ratio : Gain  Gain=Ndiff
  Divide2 : Product  Inputs=**
  Divide3 : Product  Inputs=*/
  Gear ratio look up : LookupNDDirect  NumberOfTableDimensions=1  Table=N
  Product : Product  RndMeth=Zero
  Product3 : Product  Inputs=**  RndMeth=Zero
  Switch1 : Switch  Criteria=u2 > Threshold  SaturateOnIntegerOverflow=off  InputSameDT=off
  Trans Eta : Subsystem
  neutral : Constant  Value=0
  EngTrqMaxWhls : Outport  VectorParamsAs1DForOutWhenUnconnected=off
  wires:
  Product/1 -> Product3/2
  Switch1/1 -> Diff Eta/2(TrqIn), Diff ratio/1
  Gear ratio look up/1 -> Divide3/2, Product/1
  Gear/1 -> Gear ratio look up/1, Trans Eta/3(Gear), Switch1/2
  Trans Eta/1(eta) -> Product3/1
  neutral/1 -> Switch1/3
  Product3/1 -> Switch1/1
  Diff ratio/1 -> Divide2/2
  EngSpd/1 -> [Spd], Trans Eta/2(SpdIn)
  EngTrq/1 -> Trans Eta/1(TrqIn), Product/2
  Diff Eta/1(eta) -> Divide2/1
  Divide2/1 -> EngTrqMaxWhls/1
  Divide3/1 -> Diff Eta/1(SpdIn)
  [Spd] -> Divide3/1

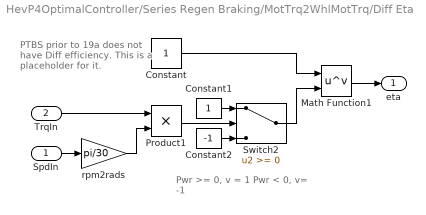
== system HevP4OptimalController/Series Regen Braking/MotTrq2WhlMotTrq/Diff Eta ==
  note: Pwr >= 0, v = 1
      | Pwr < 0, v= -1
  note: PTBS prior to 19a
      | does not have Diff
      | efficiency.  This is a
      | placeholder for it.
  SpdIn : Inport
  TrqIn : Inport  Port=2
  Constant : Constant
  Constant1 : Constant  SampleTime=-1
  Constant2 : Constant  Value=-1  SampleTime=-1
  Math Function1 : Math  Operator=pow  SignedPower=on  OutputSignalType=real
  Product1 : Product
  Switch2 : Switch  SaturateOnIntegerOverflow=off  InputSameDT=off
  rpm2rads : Gain  Gain=pi/30
  eta : Outport  VectorParamsAs1DForOutWhenUnconnected=off
  wires:
  rpm2rads/1 -> Product1/2
  Constant/1 -> Math Function1/1
  Constant2/1 -> Switch2/3
  Constant1/1 -> Switch2/1
  Product1/1 -> Switch2/2
  Switch2/1 -> Math Function1/2
  Math Function1/1 -> eta/1
  SpdIn/1 -> rpm2rads/1
  TrqIn/1 -> Product1/1

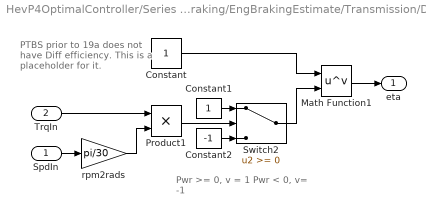
== system HevP4OptimalController/Series Regen Braking/EngBrakingEstimate/Transmission/Diff Eta ==
  note: Pwr >= 0, v = 1
      | Pwr < 0, v= -1
  note: PTBS prior to 19a
      | does not have Diff
      | efficiency.  This is a
      | placeholder for it.
  SpdIn : Inport
  TrqIn : Inport  Port=2
  Constant : Constant
  Constant1 : Constant  SampleTime=-1
  Constant2 : Constant  Value=-1  SampleTime=-1
  Math Function1 : Math  Operator=pow  SignedPower=on  OutputSignalType=real
  Product1 : Product
  Switch2 : Switch  SaturateOnIntegerOverflow=off  InputSameDT=off
  rpm2rads : Gain  Gain=pi/30
  eta : Outport  VectorParamsAs1DForOutWhenUnconnected=off
  wires:
  rpm2rads/1 -> Product1/2
  Constant/1 -> Math Function1/1
  Constant2/1 -> Switch2/3
  Constant1/1 -> Switch2/1
  Product1/1 -> Switch2/2
  Switch2/1 -> Math Function1/2
  Math Function1/1 -> eta/1
  SpdIn/1 -> rpm2rads/1
  TrqIn/1 -> Product1/1

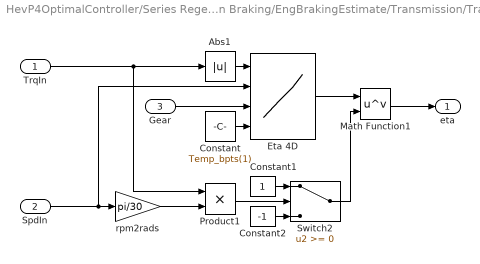
== system HevP4OptimalController/Series Regen Braking/EngBrakingEstimate/Transmission/Trans Eta ==
  TrqIn : Inport
  SpdIn : Inport  Port=2
  Gear : Inport  Port=3
  Abs1 : Abs  SaturateOnIntegerOverflow=off
  Constant : Constant  Value=Temp_bpts(1)
  Constant1 : Constant  SampleTime=-1
  Constant2 : Constant  Value=-1  SampleTime=-1
  Eta 4D : Lookup_n-D  NumberOfTableDimensions=4  LookupTableObject=''  BreakpointsForDimension1=Trq_bpts  BreakpointsForDimension2=omega_bpts  BreakpointsForDimension3=G  BreakpointsForDimension4=Temp_bpts  Table=eta_tbl  ExtrapMethod=Clip  InternalRulePriority=Speed  RndMeth=Simplest
      settings: InputPortMap=u0,u1,u2,u3
  Math Function1 : Math  Operator=pow  SignedPower=on  OutputSignalType=real
  Product1 : Product
  Switch2 : Switch  SaturateOnIntegerOverflow=off  InputSameDT=off
  rpm2rads : Gain  Gain=pi/30
  eta : Outport  VectorParamsAs1DForOutWhenUnconnected=off
  wires:
  TrqIn/1 -> Product1/1, Abs1/1
  SpdIn/1 -> Eta 4D/2, rpm2rads/1
  Math Function1/1 -> eta/1
  Abs1/1 -> Eta 4D/1
  Switch2/1 -> Math Function1/2
  Product1/1 -> Switch2/2
  Constant1/1 -> Switch2/1
  Constant2/1 -> Switch2/3
  Eta 4D/1 -> Math Function1/1
  rpm2rads/1 -> Product1/2
  Gear/1 -> Eta 4D/3
  Constant/1 -> Eta 4D/4
